simulink model "mpc_afti16"  (Simulink 6.0)
settings: Solver=ode45  SolverMode=SingleTasking  StartTime=0.0  StopTime=5  RelTol=1e-3
values from neighbouring files (symbols this model uses):
  A = sys.a    [misosim.m]    (also in misoss.m)
  B = sys.b    [misosim.m]    (also in misoss.m)
  C = sys.c    [misosim.m]    (also in misoss.m)
  D = sys.d    [misosim.m]    (also in misoss.m)
  x0 = [0 0 0 0 0]'    [misosim.m]    (also in misoss.m; mpcmotormodel.m = zeros(4,1))
libraries: mpclib x1
settings Model: Creator=jowen  LastModifiedBy=jowen  ExtModeTrigMode=oneshot  ExtModeArmWhenConnect=off
settings DataIOCC: LimitDataPoints=off  SignalLoggingName=sigsOut
settings OptimizationCC: BooleanDataType=off
settings DebuggingCC: CheckExecutionContextPreStartOutputMsg=on  CheckExecutionContextRuntimeOutputMsg=on  SolverPrmCheckMsg=none  IntegerOverflowMsg=none
settings HardwareCC: TargetUnknown=on
settings SFSimCC: SFSimApplyToAllLibs=on  SFSimBuildMode=Incremental

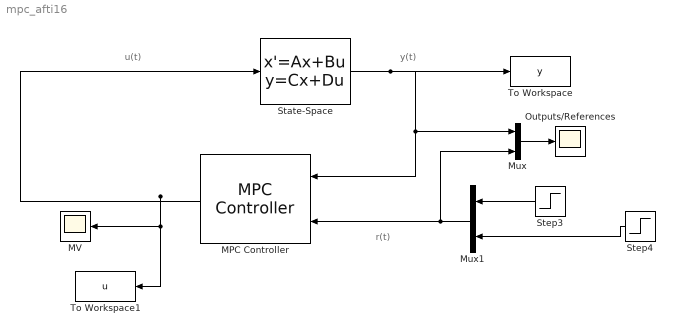
== system mpc_afti16 ==
  note: u(t)
  note: y(t)
  note: r(t)
  MPC Controller : mpclib/MPC Controller  Orientation=left  mpcobj=mpcafti  n_mv=0  x0=[]  ref_from_ws=off  ref_signal_name=[]  ref_preview=on  md_from_ws=off  md_signal_name=[]  md_preview=on  from_project=off  md_inport=off  project_file=MPCtask.mat
  MV : Scope
      settings: TimeRange=2  YMin=-20  YMax=30  DataFormat=Structure
  Mux : Mux  Inputs=2
  Mux1 : Mux  Orientation=left  Inputs=2
  Outputs/References : Scope
      settings: TimeRange=2  YMax=15  DataFormat=Structure
  State-Space : StateSpace  A=A  B=B  C=C  D=D  X0=x0
  Step3 : Step  Orientation=left  Time=0  After=0  SampleTime=0
  Step4 : Step  Orientation=left  Time=0  After=10  SampleTime=0
  To Workspace : ToWorkspace  VariableName=y  SampleTime=-1  SaveFormat=Array
  To Workspace1 : ToWorkspace  VariableName=u  SampleTime=-1  SaveFormat=Array
  wires:
  State-Space/1 -> To Workspace/1, Mux/1, MPC Controller/1
  Mux/1 -> Outputs/References/1
  MPC Controller/1 -> MV/1, To Workspace1/1, State-Space/1
  Step3/1 -> Mux1/1
  Step4/1 -> Mux1/2
  Mux1/1 -> Mux/2, MPC Controller/2
